simulink model "p2_a"  (R2017a)
settings: Solver=VariableStepAuto  StartTime=0.0  StopTime=20  RelTol=1e-3
libraries: simulink x1
settings Model: Creator=Merc  LastModifiedBy=Merc

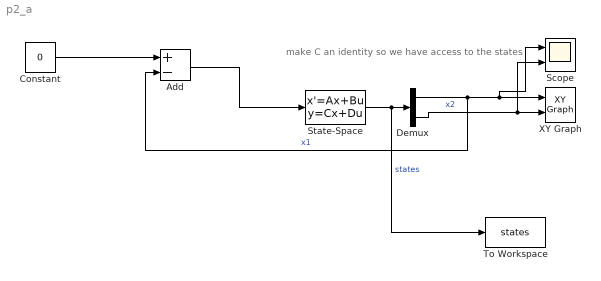
== system p2_a ==
  note: make C an identity so we have access to the states
  Add : Sum  Inputs=+-
  Constant : Constant  Value=0
  Demux : Demux  Outputs=2
  Scope : Scope  NumInputPorts=2
  State-Space : StateSpace  A=[-20, -204; 1 0]  B=[1;0]  C=eye(2)  D=[0;0]  X0=[10;10]  ContinuousStateAttributes={'x1', 'x2'}
  To Workspace : ToWorkspace  VariableName=states  SaveFormat=Timeseries  SampleTime=-1
  XY Graph : simulink/Sinks/XY Graph  xmin=-100  xmax=100  ymin=-100  ymax=100  st=-1
  wires:
  State-Space/1 -> To Workspace/1, Demux/1  "states"
  Demux/1 -> Add/2, Scope/1, XY Graph/1  "x1"
  Demux/2 -> XY Graph/2, Scope/2  "x2"
  Constant/1 -> Add/1
  Add/1 -> State-Space/1
